simulink model "ForwardKinematics"  (R2017b)
settings: Solver=VariableStepAuto  StartTime=0.0  StopTime=10.0  RelTol=1e-3
settings Model: Creator=jrv  LastModifiedBy=jrv

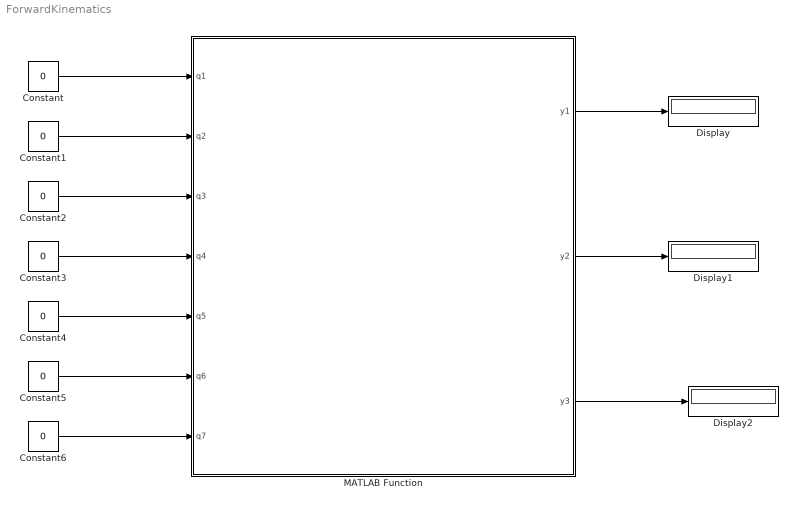
== system ForwardKinematics ==
  Constant{,1..6} (7 alike) : Constant  Value=0
  Display : Display
  Display1 : Display
  Display2 : Display
  MATLAB Function : MATLAB Function  TreatAsAtomicUnit=on
  wires:
  MATLAB Function/3(y3) -> Display2/1
  MATLAB Function/2(y2) -> Display1/1
  MATLAB Function/1(y1) -> Display/1
  Constant/1 -> MATLAB Function/1(q1)
  Constant6/1 -> MATLAB Function/7(q7)
  Constant5/1 -> MATLAB Function/6(q6)
  Constant4/1 -> MATLAB Function/5(q5)
  Constant3/1 -> MATLAB Function/4(q4)
  Constant2/1 -> MATLAB Function/3(q3)
  Constant1/1 -> MATLAB Function/2(q2)

== matlab function ForwardKinematics/MATLAB Function ==
  data: q1 input; y1 output; q2 input; q3 input; q4 input; q5 input; q6 input; q7 input; y2 output; y3 output
function [y1, y2, y3 ] = fcn( q1, q2, q3, q4, q5, q6, q7)

coder.extrinsic('SolveFK');

res = SolveFK(q1, q2, q3, q4, q5, q6, q7);
y1 = 0;
y2 = 0;
y3 = 0;
y1  = res(1) ;
y2  = res(2) ;
y3  = res(3) ;
